simulink model "xpccanpc104"  (Simulink 5.0)
settings: Solver=FixedStepDiscrete  StartTime=0.0  StopTime=300  RelTol=1e-3
undefined symbols (not defined in the file or in its folder): bit, Standard
libraries: xpclib x6
settings Model: Creator=mvetsch  LastModifiedBy=ekbas  ExtModeMexFile=ext_xpc  ExtModeArmWhenConnect=off  SignalLoggingName=logsOut  BlockReductionOpt=off  BooleanDataType=off  OptimizeBlockIOStorage=off  ZeroCrossControl=UseLocalSettings  TargetHWChar=2  TargetHWWordLengths=8,16,32,32  RTWSystemTargetFile=xpctarget.tlc  RTWTemplateMakefile=xpc_default_tmf  RTWMathFcnLibMatFile=iso_c_tmw.mat  RTWOptions="-aEnforceIntegerDowncast=1 -aFoldNonRolledExpr=1 -aInlineInvariantSignals=0 -aInlineParameters=0 -aLocalBlockOutputs=0 -aRollThreshold=5 -aGenerateReport=0 -aGenCodeOnly=0 -aRTWVerbose=1 -aForceParamTrailComments=0 -aGenerateComments=1 -aIgnoreCustomStorageClasses=1 -aIncHierarchyInIds=0 -aMaxRTWIdLen=31 -aShowEliminatedStatements=1 -aPrefixModelToSubsysFcnNames=1 -aIncDataTypeInIds=0 -aInlinedPrmAccess=\"Literals\" -aTargetFcnLib=\"iso_c_tmw.mat\" -aGenerateFullHeader=1 -aIsPILTarget=0 -aRL32ModeModifier=\"Real-Time\" -aRL32LogTETModifier=1 -aRL32LogBufSizeModifier=100000 -aRL32IRQSourceModifier=\"Timer\" -axPCIRQSourceBoard=\"None/Other\" -axPCIOIRQSlot=-1 -aLocalBlockOutputs=0 -axpcDblBuff=0 -axpcObjCom=0 -aRL32ObjectName=\"tg\" -aExtMode=1 -aRL32ScopeModifier=1"

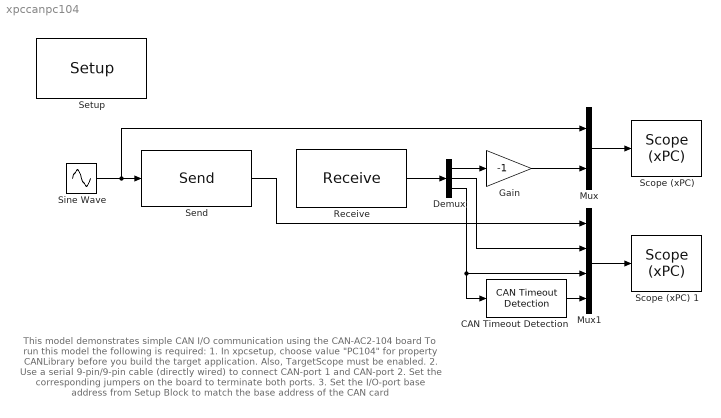
== system xpccanpc104 ==
  note: This model demonstrates simple CAN I/O communication using the CAN-AC2-104 board
      |
      | To run this model the following is required:
      |
      | 1. In xpcsetup, choose value "PC104" for property CANLibrary before you build the
      | target application. Also, TargetScope must be enabled.
      |
      | 2. Use a serial 9-pin/9-pin cable (directly wired) to connect CAN-port 1 and CAN-port 2.
      | Set the corresponding jumpers on the board to terminate both ports.
      |
      | 3. Set the I/O-port base address from Setup Block  to match the base address of the CAN card
  CAN Timeout Detection : xpclib/CAN/Utilities/CAN Timeout Detection  timeout=0.02
  Demux : Demux  Outputs=3
  Gain : Gain  Gain=-1  SaturateOnIntegerOverflow=on
  Mux : Mux  Inputs=2
  Mux1 : Mux
  "Receive " : xpclib/CAN/Softing/CAN-AC2-104 SJA 1000/Receive   board=1  canPort=CAN 2  range=Standard (11-bit)  ids=[50]  output=Data - Status - Timestamp  inten=off  ts=0.01  ididx=[0]
  "Scope (xPC) " : xpclib/Misc./Scope (xPC)   scopeno=1  scopetype=Target  autostart=on  viewmode=Graphical rolling  formatstr='%15.6f'  grid=on  ylimits=[0,0]  nosamples=250  noprepostsamples=0  interleave=1  triggermode=FreeRun  triggersignal=1  triggerlevel=0.0  triggerslope=Either  triggerscope=1  triggersample=0  filename=data.dat  mode=Lazy  writesize=512  autorestart=off
  Scope (xPC) 1 : xpclib/Misc./Scope (xPC)   scopeno=2  scopetype=Target  autostart=on  viewmode=Numerical  formatstr='%15.6f'  grid=on  ylimits=[0,0]  nosamples=10  noprepostsamples=0  interleave=1  triggermode=FreeRun  triggersignal=1  triggerlevel=0.0  triggerslope=Either  triggerscope=1  triggersample=0  filename=data.dat  mode=Lazy  writesize=512  autorestart=off
  "Send " : xpclib/CAN/Softing/CAN-AC2-104 SJA 1000/Send   board=1  canPort=CAN 1  range=Standard (11-bit)  ids=[50]  sizes=[8]  output=on  ts=0.01  ididx=[0]
  "Setup " : xpclib/CAN/Softing/CAN-AC2-104 SJA 1000/Setup   board=1  can1Baudrate=1 MBaud  can1UserBR=[1,1,4,3]  can2Baudrate=1 MBaud  can2UserBR=[1,1,4,3]  init=[]  term=[]  ioBaseAddressL=0x300  memBaseAddressL=0xd0000  intNo=None
  Sine Wave : Sin  Frequency=5  SampleTime=0.01
  wires:
  Sine Wave/1 -> "Send "/1, Mux/1
  "Receive "/1 -> Demux/1
  Demux/1 -> Gain/1
  Gain/1 -> Mux/2
  Mux/1 -> "Scope (xPC) "/1
  Mux1/1 -> Scope (xPC) 1/1
  Demux/3 -> Mux1/3, CAN Timeout Detection/1
  Demux/2 -> Mux1/2
  CAN Timeout Detection/1 -> Mux1/4
  "Send "/1 -> Mux1/1
